simulink model "vexv5_Replay_Motion"  (R2019b)
settings: Solver=ode3  StartTime=0.0  StopTime=20  RelTol=1e-3  EnableMultiTasking=on
libraries: vexv5lib x4, vexv5_SD_Logging_Lib x1
settings Model: SimulationMode=external  ExtModeTrigDuration=5  Creator=The MathWorks, Inc.  LastModifiedBy=josea
settings DataIOCC: LimitDataPoints=on  SaveFormat=Array  ReturnWorkspaceOutputs=off
settings OptimizationCC: ExpressionDepthLimit=2147483647  LifeSpan=Inf  MaxStackSize=64  EfficientTunableParamExpr=on
settings DebuggingCC: UnderspecifiedInitializationDetection=Classic  MergeDetectMultiDrivingBlocksExec=none  InheritedTsInSrcMsg=none  FcnCallInpInsideContextMsg=warning  UnconnectedInputMsg=none  UnconnectedOutputMsg=none  AllowSymbolicDim=off  StateNameClashWarn=warning  SFUnexpectedBacktrackingDiag=warning  SFNoUnconditionalDefaultTransitionDiag=warning  SFExecutionAtInitializationDiag=none  ArithmeticOperatorsInVariantConditions=warning
settings HardwareCC: ProdBitPerPointer=32  ProdBitPerSizeT=32  ProdBitPerPtrDiffT=32  ProdLargestAtomicInteger=Long  ProdLargestAtomicFloat=Double  ProdWordSize=32  ProdHWDeviceType=ARM Compatible->ARM Cortex
settings ModelReferenceCC: PropagateSignalLabelsOutOfModel=off
settings SFSimCC: SimUseLocalCustomCode=off  CustomCodeUndefinedFunction=UseInterfaceOnly
settings RTWCC: SystemTargetFile=ert.tlc  HardwareBoard=VEX V5 Robot Brain  TLCOptions=-aInlineSetEventsForThisBaseRateFcn=TLC_FALSE -aSuppressMultiTaskScheduler=TLC_FALSE -aRateBasedStepFcn=0  TemplateMakefile=ert_default_tmf  RTWUseLocalCustomCode=off  Toolchain=GNU Tools for ARM Embedded Processors
settings CodeAppCC: StateflowObjectComments=on
settings ERTTargetCC: CodeReplacementLibrary=GCC ARM Cortex-M3  MultiwordLength=2048  ERTCustomFileBanners=off  MatFileLogging=on  SupportContinuousTime=on  SupportNonInlinedSFcns=on  RemoveResetFunc=off  ModelStepFunctionPrototypeControlCompliant=off  ConvertIfToSwitch=off  SuppressUnreachableDefaultCases=off
settings ConfigComp: CovMetricSettings=dw  CovHtmlReporting=on  CovSaveCumulativeToWorkspaceVar=on  CovSaveSingleToWorkspaceVar=on  CovExternalEMLEnable=off  CovSFcnEnable=off

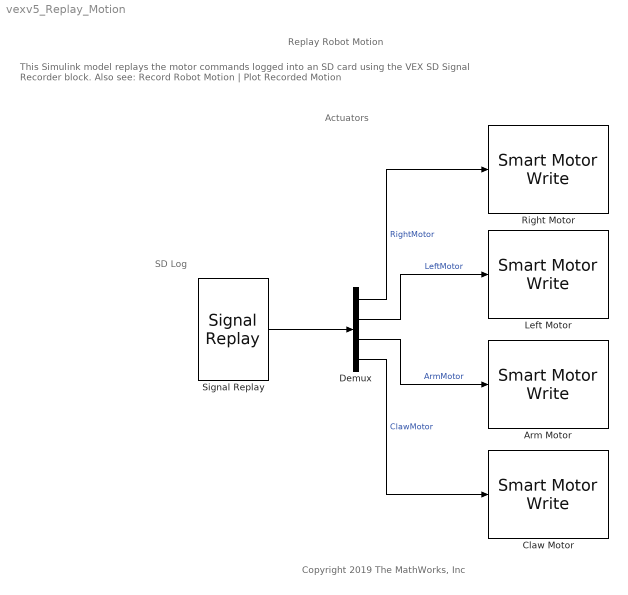
== system vexv5_Replay_Motion ==
  note: SD Log
  note: Actuators
  note: Copyright 2019 The MathWorks, Inc
  note: Replay Robot Motion
  note: This Simulink model replays the motor commands logged into an SD card using the VEX SD Signal Recorder block.
      | Also see: Record Robot Motion | Plot Recorded Motion
  Arm Motor : vexv5lib/Actuators/Smart Motor Write  motorPort=8  scaleFactor=18:1  MotorBrakeMode=Hold  OperationMode=Velocity Control
      settings: SourceProductName=Simulink Coder Support Package for VEX EDR V5 Robot Brain
  Claw Motor : vexv5lib/Actuators/Smart Motor Write  motorPort=3  scaleFactor=18:1  MotorBrakeMode=Hold  OperationMode=Velocity Control
      settings: SourceProductName=Simulink Coder Support Package for VEX EDR V5 Robot Brain
  Demux : Demux
  Left Motor : vexv5lib/Actuators/Smart Motor Write  motorPort=1  scaleFactor=18:1  MotorBrakeMode=Coast  OperationMode=Velocity Control
      settings: SourceProductName=Simulink Coder Support Package for VEX EDR V5 Robot Brain
  Right Motor : vexv5lib/Actuators/Smart Motor Write  motorPort=10  scaleFactor=18:1  MotorBrakeMode=Coast  OperationMode=Velocity Control
      settings: SourceProductName=Simulink Coder Support Package for VEX EDR V5 Robot Brain
  Signal Replay : vexv5_SD_Logging_Lib/Signal Replay  sel_session=vexv5_Right_Turn_1__stitched
  wires:
  Signal Replay/1 -> Demux/1
  Demux/1 -> Right Motor/1  "RightMotor"
  Demux/2 -> Left Motor/1  "LeftMotor"
  Demux/3 -> Arm Motor/1  "ArmMotor"
  Demux/4 -> Claw Motor/1  "ClawMotor"
